simulink model "InvertedPendulum_REV0"  (R2018a)
settings: Solver=VariableStepAuto  StartTime=0.0  StopTime=T_STOP  RelTol=1e-3
values from neighbouring files (symbols this model uses):
  A_dist = 0    [InvertedPendulum.m]    (also in InvertedPendulumStepResponse.m)
  Ac = [0 1 0 0 ... (first row only)    [BasicModelParameters.m]    (also in ControllerDesign_REV0.m; FurutaPendulum.m = [0 1 0 0; 0 0 -a23 0; 0 0 0 1; 0 0 a43 0]; InvertedPendulumStepResponse.m)
  Bc = transpose([0 b21 0 -b41])    [BasicModelParameters.m]    (also in ControllerDesign_REV0.m; FurutaPendulum.m = [0; b21; 0; -b41]; InvertedPendulumStepResponse.m)
  Cc = [1 0 0 0 ... (first row only)    [BasicModelParameters.m]    (also in ControllerDesign_REV0.m; FurutaPendulum.m = [1 0 0 0; 0 0 1 0]; InvertedPendulumStepResponse.m)
  Dc = [0 ... (first row only)    [BasicModelParameters.m]    (also in ControllerDesign_REV0.m; FurutaPendulum.m = [0; 0]; InvertedPendulumStepResponse.m)
  f_dist = 10    [InvertedPendulum.m]    (also in InvertedPendulumStepResponse.m)
  k1 = [-5.2947]    [InvertedPendulum.m]    (also in InvertedPendulumStepResponse.m)
  k2 = [-5.1415]    [InvertedPendulum.m]    (also in InvertedPendulumStepResponse.m)
  p1 = [-284.8, 0]    [InvertedPendulum.m]    (also in InvertedPendulumStepResponse.m)
  p2 = [-50]    [InvertedPendulum.m]    (also in InvertedPendulumStepResponse.m)
  theta1_cmd_A = pi/4    (= 0.785398163397)    [InvertedPendulum.m]    (also in InvertedPendulumStepResponse.m)
  theta1_cmd_f = 0.1    [InvertedPendulum.m]    (also in InvertedPendulumStepResponse.m)
  z1 = [-0.1229, -0.02181]    [InvertedPendulum.m]    (also in InvertedPendulumStepResponse.m)
  z2 = [-9.249]    [InvertedPendulum.m]    (also in InvertedPendulumStepResponse.m)
settings Model: Creator=Jack  LastModifiedBy=Jack

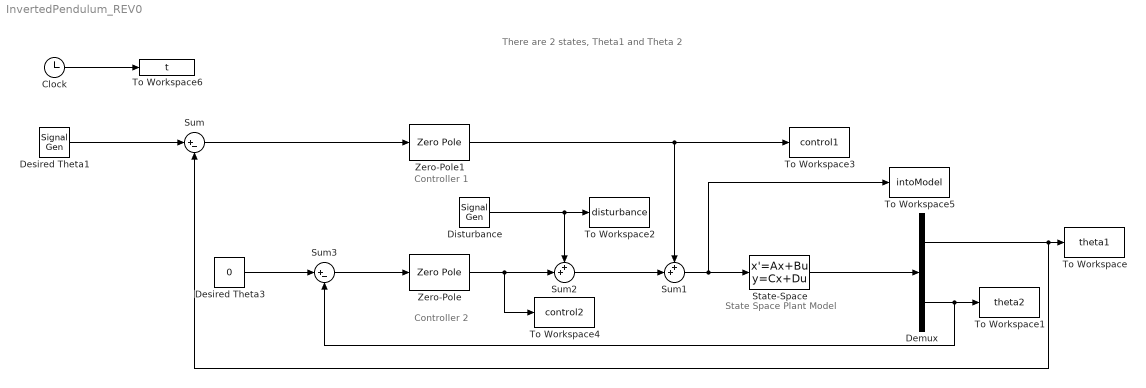
== system InvertedPendulum_REV0 ==
  note: Controller 1
  note: There are 2 states, Theta1 and Theta 2
  note: State Space Plant Model
  note: Controller 2
  Clock : Clock
  Demux : Demux  Outputs=2
  Desired Theta3 : Constant  Value=0
  Desired Theta1 : SignalGenerator  Amplitude=theta1_cmd_A  Frequency=theta1_cmd_f
  "Disturbance " : SignalGenerator  Amplitude=A_dist  Frequency=f_dist
  State-Space : StateSpace  A=Ac  B=Bc  C=Cc  D=Dc  InitialCondition=[0; 0; 0.05; 0]  ContinuousStateAttributes='Theta'
  Sum : Sum  Inputs=|+-
  Sum1 : Sum  Inputs=++|
  Sum2 : Sum  Inputs=++|
  Sum3 : Sum  Inputs=|+-
  To Workspace : ToWorkspace  VariableName=theta1  SampleTime=-1
  To Workspace1 : ToWorkspace  VariableName=theta2  SampleTime=-1
  To Workspace2 : ToWorkspace  VariableName=disturbance  SampleTime=-1
  To Workspace3 : ToWorkspace  VariableName=control1  SampleTime=-1
  To Workspace4 : ToWorkspace  VariableName=control2  SampleTime=-1
  To Workspace5 : ToWorkspace  VariableName=intoModel  SampleTime=-1
  To Workspace6 : ToWorkspace  VariableName=t  SampleTime=-1
  Zero-Pole : ZeroPole  Zeros=z2  Poles=p2  Gain=k2
  Zero-Pole1 : ZeroPole  Zeros=z1  Poles=p1  Gain=k1
  wires:
  Desired Theta1/1 -> Sum/1
  Sum/1 -> Zero-Pole1/1
  State-Space/1 -> Demux/1
  Sum1/1 -> To Workspace5/1, State-Space/1
  Demux/1 -> Sum/2, To Workspace/1
  Demux/2 -> Sum3/2, To Workspace1/1
  Desired Theta3/1 -> Sum3/1
  Zero-Pole/1 -> To Workspace4/1, Sum2/2
  Sum3/1 -> Zero-Pole/1
  "Disturbance "/1 -> Sum2/1, To Workspace2/1
  Sum2/1 -> Sum1/2
  Zero-Pole1/1 -> To Workspace3/1, Sum1/1
  Clock/1 -> To Workspace6/1
